simulink model "Vorlage_Anlagenteil_Pruefen_Jaehocha"  (R2021b)
settings: Solver=ode3  StartTime=0.0  StopTime=50  FixedStep=0.01  RelTol=1e-3
StopFcn:
  | clear con
model workspace (MAT data in the model file):
  A = Simulink.Signal
  A.DataType = 'auto'
  A.Dimensions = 1
  A.DimensionsMode = 'auto'
  A.Complexity = 'auto'
  A.SampleTime = -1
  A.SamplingMode = 'auto'
undefined symbols (not defined in the file): sigbuilder_block
libraries: simulink x10, simulink_extras x7, aerolibanimutils x1
(part 1 of 2)
settings Model: Creator=Jan  LastModifiedBy=mwjae
settings SolverCC: AlgebraicLoopSolver=TrustRegion
settings DataIOCC: ReturnWorkspaceOutputs=off
settings DebuggingCC: SFMachineParentedDataDiag=warning  ArithmeticOperatorsInVariantConditions=warning
settings SFSimCC: SimUseLocalCustomCode=off  CustomCodeUndefinedFunction=UseInterfaceOnly
settings RTWCC: RTWUseLocalCustomCode=off
settings CodeAppCC: StateflowObjectComments=on
settings SimscapeCC: SimscapeNormalizeSystem=off

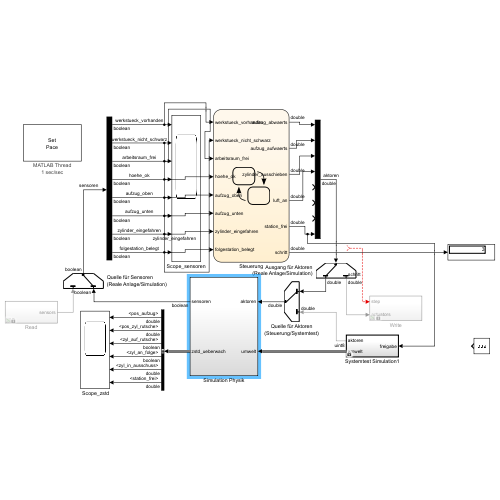
[thumbnail: Simulink's stored preview of the top-level diagram]
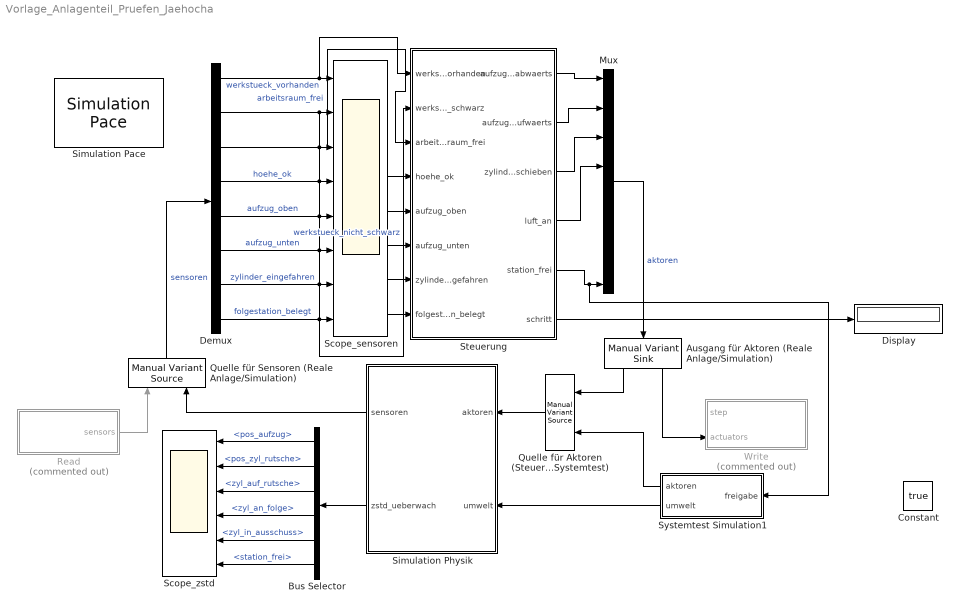
== system Vorlage_Anlagenteil_Pruefen_Jaehocha ==
  " Scope_zstd" : Scope  NumInputPorts=6
  Ausgang für Aktoren (Reale Anlage/Simulation) : simulink/Signal Routing/Manual Variant Sink  NumChoices=2  LabelModeActiveChoice=V_1
  Bus Selector : BusSelector  OutputSignals=pos_aufzug,pos_zyl_rutsche,zyl_auf_rutsche,zyl_an_folge,zyl_in_ausschuss,station_frei
  Constant : Constant  Value=true
  Demux : Demux  Outputs=8
  Display : Display
  Mux : Mux  Inputs=8
  Quelle für Aktoren (Steuerung/Systemtest) : simulink/Signal Routing/Manual Variant Source  NumChoices=2  LabelModeActiveChoice=V_1
  Quelle für Sensoren (Reale Anlage/Simulation) : simulink/Signal Routing/Manual Variant Source  NumChoices=2  LabelModeActiveChoice=V_2
  Read : Subsystem  Commented=on
  Scope_sensoren : Scope  NumInputPorts=8
  Simulation Pace : aerolibanimutils/Simulation Pace  SimulationPace=1  SleepMode=MATLAB Thread  OutputPaceError=off  SampleTime=-1
  Simulation Physik : Subsystem
  Steuerung : Stateflow chart  TreatAsAtomicUnit=on
  Systemtest Simulation1 : Subsystem  TreatAsAtomicUnit=on
  Write : Subsystem  Commented=on
  wires:
  Quelle für Sensoren (Reale Anlage/Simulation)/1 -> Demux/1  "sensoren"
  Read/1(sensors) -> Quelle für Sensoren (Reale Anlage/Simulation)/1
  Mux/1 -> Ausgang für Aktoren (Reale Anlage/Simulation)/1  "aktoren"
  Simulation Physik/1(sensoren) -> Quelle für Sensoren (Reale Anlage/Simulation)/2
  Ausgang für Aktoren (Reale Anlage/Simulation)/2 -> Write/2(actuators)
  Ausgang für Aktoren (Reale Anlage/Simulation)/1 -> Quelle für Aktoren (Steuerung/Systemtest)/1
  Quelle für Aktoren (Steuerung/Systemtest)/1 -> Simulation Physik/1(aktoren)
  Systemtest Simulation1/1(aktoren) -> Quelle für Aktoren (Steuerung/Systemtest)/2
  Systemtest Simulation1/2(umwelt) -> Simulation Physik/2(umwelt)
  Simulation Physik/2(zstd_ueberwach) -> Bus Selector/1
  Bus Selector/1 -> " Scope_zstd"/1  "<pos_aufzug>"
  Bus Selector/2 -> " Scope_zstd"/2  "<pos_zyl_rutsche>"
  Bus Selector/3 -> " Scope_zstd"/3  "<zyl_auf_rutsche>"
  Bus Selector/4 -> " Scope_zstd"/4  "<zyl_an_folge>"
  Bus Selector/5 -> " Scope_zstd"/5  "<zyl_in_ausschuss>"
  Bus Selector/6 -> " Scope_zstd"/6  "<station_frei>"
  Demux/1 -> Steuerung/1(werkstueck_vorhanden), Scope_sensoren/1  "werkstueck_vorhanden"
  Demux/2 -> Steuerung/2(werkstueck_nicht_schwarz), Scope_sensoren/2  "werkstueck_nicht_schwarz"
  Demux/3 -> Steuerung/3(arbeitsraum_frei), Scope_sensoren/3  "arbeitsraum_frei"
  Demux/4 -> Scope_sensoren/4, Steuerung/4(hoehe_ok)  "hoehe_ok"
  Demux/5 -> Steuerung/5(aufzug_oben), Scope_sensoren/5  "aufzug_oben"
  Demux/6 -> Steuerung/6(aufzug_unten), Scope_sensoren/6  "aufzug_unten"
  Demux/7 -> Steuerung/7(zylinder_eingefahren), Scope_sensoren/7  "zylinder_eingefahren"
  Demux/8 -> Steuerung/8(folgestation_belegt), Scope_sensoren/8  "folgestation_belegt"
  ? -> Write/1(step)  "schritt"
  Steuerung/5(station_frei) -> Systemtest Simulation1/1(freigabe), Mux/8
  Steuerung/1(aufzug_abwaerts) -> Mux/1
  Steuerung/2(aufzug_aufwaerts) -> Mux/2
  Steuerung/3(zylinder_ausschieben) -> Mux/3
  Steuerung/4(luft_an) -> Mux/4
  Steuerung/6(schritt) -> Display/1

== system Vorlage_Anlagenteil_Pruefen_Jaehocha/Read ==
  Read : MATLAB Function  TreatAsAtomicUnit=on
  sensors : Outport  VectorParamsAs1DForOutWhenUnconnected=off
  wires:
  Read/1(senarr) -> sensors/1

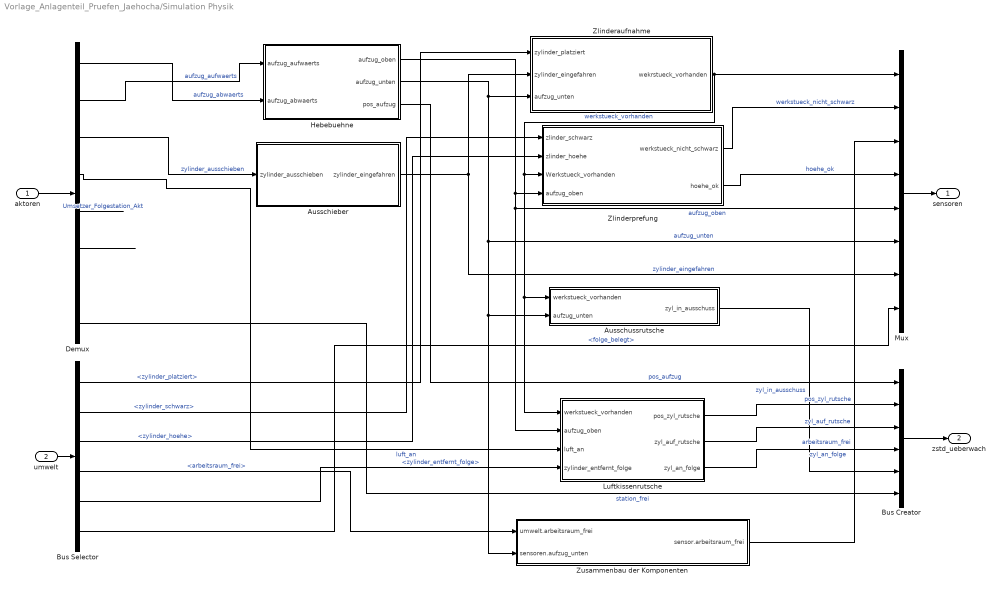
== system Vorlage_Anlagenteil_Pruefen_Jaehocha/Simulation Physik ==
  aktoren : Inport
  umwelt : Inport  Port=2
  Ausschieber : Subsystem
  Ausschussrutsche : Subsystem
  Bus Creator : BusCreator  Inputs=6
  Bus Selector : BusSelector  OutputSignals=zylinder_platziert,zylinder_schwarz,zylinder_hoehe,arbeitsraum_frei,zylinder_entfernt_folge,folge_belegt
  Demux : Demux  Outputs=8
  Hebebuehne : Subsystem
  Luftkissenrutsche : Subsystem
  Mux : Mux  Inputs=8
  Zlinderaufnahme : Subsystem
  Zlinderprefung : Subsystem
  Zusammenbau der Komponenten : Subsystem
  sensoren : Outport  VectorParamsAs1DForOutWhenUnconnected=off
  zstd_ueberwach : Outport  Port=2  VectorParamsAs1DForOutWhenUnconnected=off
  wires:
  aktoren/1 -> Demux/1
  Mux/1 -> sensoren/1
  Zusammenbau der Komponenten/1(sensor.arbeitsraum_frei) -> Mux/3  "arbeitsraum_frei"
  Demux/3 -> Ausschieber/1(zylinder_ausschieben)  "zylinder_ausschieben"
  Zlinderaufnahme/1(wekrstueck_vorhanden) -> Ausschussrutsche/1(werkstueck_vorhanden), Luftkissenrutsche/1(werkstueck_vorhanden), Zlinderprefung/3(Werkstueck_vorhanden), Mux/1  "werkstueck_vorhanden"
  Zlinderprefung/2(hoehe_ok) -> Mux/4  "hoehe_ok"
  Zlinderprefung/1(werkstueck_nicht_schwarz) -> Mux/2  "werkstueck_nicht_schwarz"
  umwelt/1 -> Bus Selector/1
  Bus Selector/2 -> Zlinderprefung/1(zlinder_schwarz)  "<zylinder_schwarz>"
  Bus Selector/4 -> Zusammenbau der Komponenten/1(umwelt.arbeitsraum_frei)  "<arbeitsraum_frei>"
  Bus Selector/5 -> Luftkissenrutsche/4(zylinder_entfernt_folge)  "<zylinder_entfernt_folge>"
  Bus Selector/6 -> Mux/8  "<folge_belegt>"
  Hebebuehne/3(pos_aufzug) -> Bus Creator/1  "pos_aufzug"
  Bus Creator/1 -> zstd_ueberwach/1
  Luftkissenrutsche/1(pos_zyl_rutsche) -> Bus Creator/2  "pos_zyl_rutsche"
  Luftkissenrutsche/2(zyl_auf_rutsche) -> Bus Creator/3  "zyl_auf_rutsche"
  Luftkissenrutsche/3(zyl_an_folge) -> Bus Creator/4  "zyl_an_folge"
  Ausschussrutsche/1(zyl_in_ausschuss) -> Bus Creator/5  "zyl_in_ausschuss"
  Hebebuehne/2(aufzug_unten) -> Mux/6, Zusammenbau der Komponenten/2(sensoren.aufzug_unten), Ausschussrutsche/2(aufzug_unten), Zlinderaufnahme/3(aufzug_unten)  "aufzug_unten"
  Ausschieber/1(zylinder_eingefahren) -> Zlinderaufnahme/2(zylinder_eingefahren), Mux/7  "zylinder_eingefahren"
  Hebebuehne/1(aufzug_oben) -> Zlinderprefung/4(aufzug_oben), Mux/5, Luftkissenrutsche/2(aufzug_oben)  "aufzug_oben"
  Bus Selector/3 -> Zlinderprefung/2(zlinder_hoehe)  "<zylinder_hoehe>"
  Demux/8 -> Bus Creator/6  "station_frei"
  Demux/1 -> Hebebuehne/2(aufzug_abwaerts)  "aufzug_abwaerts"
  Demux/2 -> Hebebuehne/1(aufzug_aufwaerts)  "aufzug_aufwaerts"
  Bus Selector/1 -> Zlinderaufnahme/1(zylinder_platziert)  "<zylinder_platziert>"
  Demux/4 -> Luftkissenrutsche/3(luft_an)  "luft_an"
  Demux/5 -> ?  "Umsetzer_Folgestation_Akt"
  Demux/6 -> ?

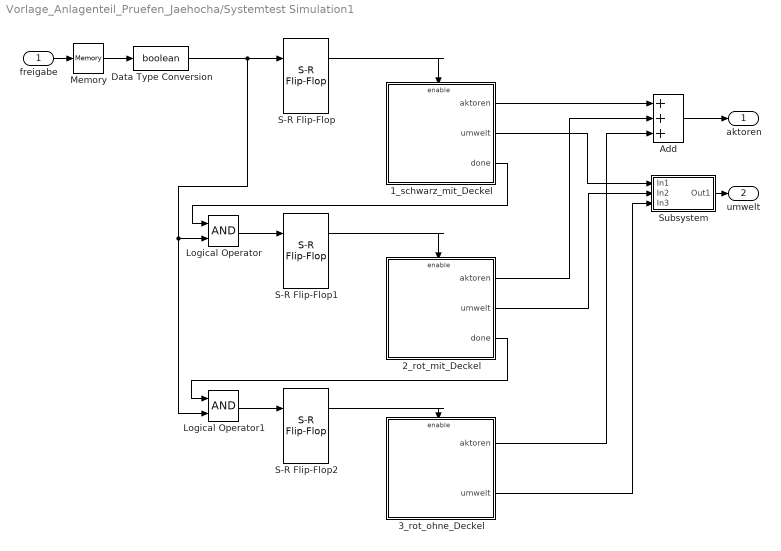
== system Vorlage_Anlagenteil_Pruefen_Jaehocha/Systemtest Simulation1 ==
  freigabe : Inport
  1_schwarz_mit_Deckel : Subsystem
  2_rot_mit_Deckel : Subsystem
  3_rot_ohne_Deckel : Subsystem
  Add : Sum  Inputs=+++
  Data Type Conversion : DataTypeConversion  OutDataTypeStr=boolean
  Logical Operator : Logic  AllPortsSameDT=off  OutDataTypeStr=boolean
  Logical Operator1 : Logic  AllPortsSameDT=off  OutDataTypeStr=boolean
  Memory : Memory
  S-R Flip-Flop : simulink_extras/Flip Flops/S-R Flip-Flop  initial_condition=0
  S-R Flip-Flop1 : simulink_extras/Flip Flops/S-R Flip-Flop  initial_condition=0
  S-R Flip-Flop2 : simulink_extras/Flip Flops/S-R Flip-Flop  initial_condition=0
  Subsystem : Subsystem
  aktoren : Outport  VectorParamsAs1DForOutWhenUnconnected=off
  umwelt : Outport  Port=2  VectorParamsAs1DForOutWhenUnconnected=off
  wires:
  freigabe/1 -> Memory/1
  S-R Flip-Flop/1 -> 1_schwarz_mit_Deckel/Enable
  Logical Operator/1 -> S-R Flip-Flop1/1
  1_schwarz_mit_Deckel/3(done) -> Logical Operator/1
  S-R Flip-Flop1/1 -> 2_rot_mit_Deckel/Enable
  Logical Operator1/1 -> S-R Flip-Flop2/1
  2_rot_mit_Deckel/3(done) -> Logical Operator1/1
  S-R Flip-Flop2/1 -> 3_rot_ohne_Deckel/Enable
  1_schwarz_mit_Deckel/1(aktoren) -> Add/1
  2_rot_mit_Deckel/1(aktoren) -> Add/2
  Add/1 -> aktoren/1
  3_rot_ohne_Deckel/1(aktoren) -> Add/3
  Subsystem/1(Out1) -> umwelt/1
  1_schwarz_mit_Deckel/2(umwelt) -> Subsystem/1(In1)
  2_rot_mit_Deckel/2(umwelt) -> Subsystem/2(In2)
  3_rot_ohne_Deckel/2(umwelt) -> Subsystem/3(In3)
  Data Type Conversion/1 -> Logical Operator1/2, Logical Operator/2, S-R Flip-Flop/1
  Memory/1 -> Data Type Conversion/1

== system Vorlage_Anlagenteil_Pruefen_Jaehocha/Write ==
  step : Inport
  actuators : Inport  Port=2
  Data Type Conversion : DataTypeConversion  OutDataTypeStr=boolean
  Write1 : MATLAB Function  TreatAsAtomicUnit=on
  wires:
  step/1 -> Write1/1(step)
  Data Type Conversion/1 -> Write1/2(actuators)
  actuators/1 -> Data Type Conversion/1

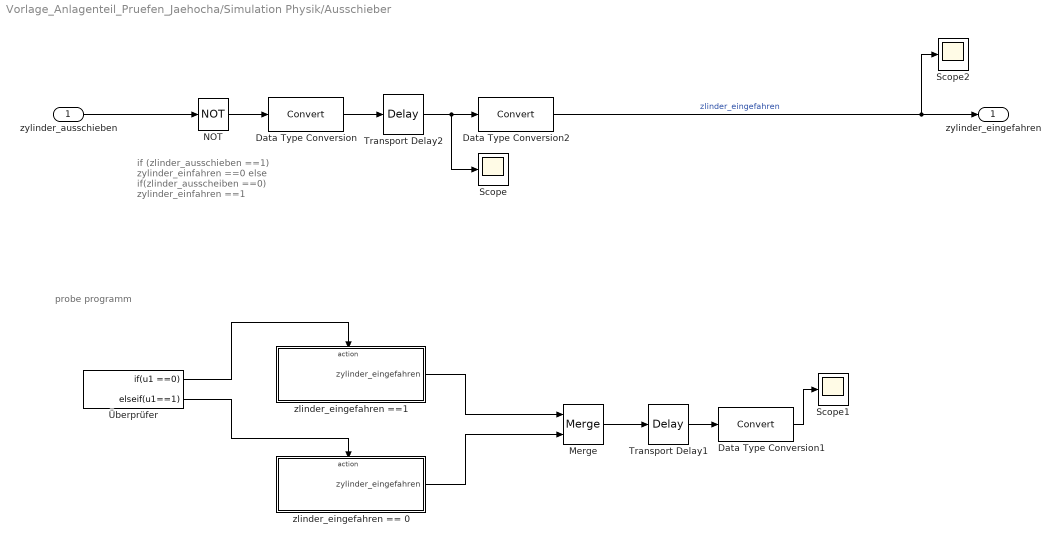
== system Vorlage_Anlagenteil_Pruefen_Jaehocha/Simulation Physik/Ausschieber ==
  note: probe programm
  note: if (zlinder_ausschieben ==1)
      |  zylinder_einfahren ==0
      | else if(zlinder_ausscheiben ==0)
      | zylinder_einfahren ==1
  zylinder_ausschieben : Inport
  Data Type Conversion : DataTypeConversion
  Data Type Conversion1 : DataTypeConversion
  Data Type Conversion2 : DataTypeConversion
  Merge : Merge
  NOT : Logic  Operator=NOT  IconShape=distinctive  AllPortsSameDT=off  OutDataTypeStr=boolean
  Scope : Scope
  Scope1 : Scope
  Scope2 : Scope
  Transport Delay1 : TransportDelay  DelayTime=0.5
  Transport Delay2 : TransportDelay  DelayTime=0.5
  zlinder_eingefahren == 0 : Subsystem  TreatAsAtomicUnit=on
  zlinder_eingefahren ==1 : Subsystem  TreatAsAtomicUnit=on
  Überprüfer : If  IfExpression=u1 ==0  ElseIfExpressions=u1==1  ShowElse=off
  zylinder_eingefahren : Outport
  wires:
  Data Type Conversion/1 -> Transport Delay2/1
  NOT/1 -> Data Type Conversion/1
  Transport Delay2/1 -> Data Type Conversion2/1, Scope/1
  zylinder_ausschieben/1 -> NOT/1
  Data Type Conversion2/1 -> zylinder_eingefahren/1, Scope2/1  "zlinder_eingefahren"
  Data Type Conversion1/1 -> Scope1/1
  zlinder_eingefahren ==1/1(zylinder_eingefahren) -> Merge/1
  Transport Delay1/1 -> Data Type Conversion1/1
  Überprüfer/2 -> zlinder_eingefahren == 0/Action
  zlinder_eingefahren == 0/1(zylinder_eingefahren) -> Merge/2
  Merge/1 -> Transport Delay1/1
  Überprüfer/1 -> zlinder_eingefahren ==1/Action

== system Vorlage_Anlagenteil_Pruefen_Jaehocha/Simulation Physik/Ausschussrutsche ==
  werkstueck_vorhanden : Inport
  aufzug_unten : Inport  Port=2
  AND : Logic  IconShape=distinctive  AllPortsSameDT=off  OutDataTypeStr=boolean
  Relational Operator : RelationalOperator  Operator=<  OutDataTypeStr=boolean  RndMeth=Simplest
  Scope : Scope  NumInputPorts=4
  Scope1 : Scope
  Triggered Subsystem for Rising edge counter : Subsystem  TreatAsAtomicUnit=on
  Unit Delay : UnitDelay  SampleTime=-1  HasFrameUpgradeWarning=on
  zyl_in_ausschuss : Outport
  wires:
  werkstueck_vorhanden/1 -> Unit Delay/1, Scope/1, Relational Operator/1  "werkstueck_vorhanden"
  aufzug_unten/1 -> Scope/3, AND/2  "aufzug_unten"
  Unit Delay/1 -> Relational Operator/2
  Relational Operator/1 -> Scope/2, AND/1  "falling Edge"
  AND/1 -> Triggered Subsystem for Rising edge counter/Trigger, Scope/4  "AND"
  Triggered Subsystem for Rising edge counter/1(zyl_in_ausschuss) -> Scope1/1, zyl_in_ausschuss/1  "zyl_in_ausschuss"

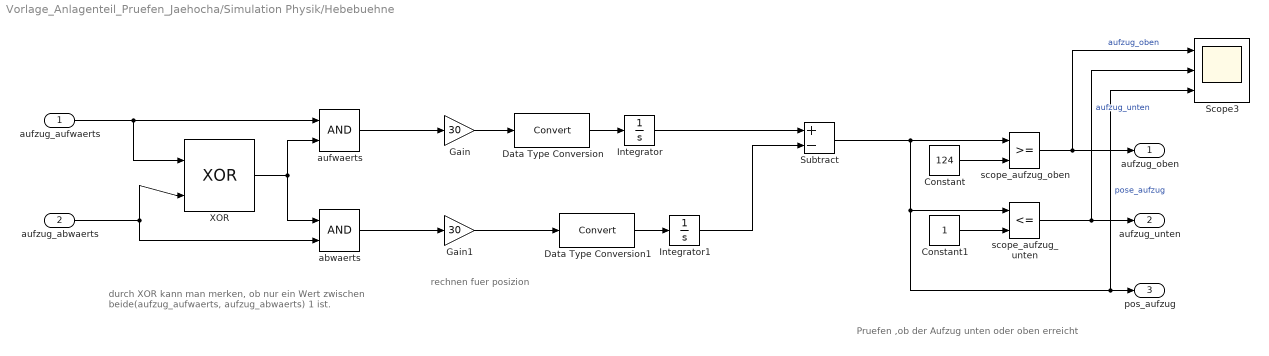
== system Vorlage_Anlagenteil_Pruefen_Jaehocha/Simulation Physik/Hebebuehne ==
  note: rechnen fuer posizion
  note: durch XOR kann man merken, ob nur ein Wert zwischen beide(aufzug_aufwaerts, aufzug_abwaerts) 1 ist.
  note: Pruefen ,ob der Aufzug unten oder oben erreicht
  aufzug_aufwaerts : Inport
  aufzug_abwaerts : Inport  Port=2
  Constant : Constant  Value=124
  Constant1 : Constant
  Data Type Conversion : DataTypeConversion
  Data Type Conversion1 : DataTypeConversion
  Gain : Gain  Gain=30
  Gain1 : Gain  Gain=30
  Integrator : Integrator  UpperSaturationLimit=125  LowerSaturationLimit=0
  Integrator1 : Integrator  UpperSaturationLimit=0  LowerSaturationLimit=-125
  Scope3 : Scope  NumInputPorts=3
  Subtract : Sum  Inputs=+-
  XOR : Logic  Operator=XOR  IconShape=distinctive  AllPortsSameDT=off  OutDataTypeStr=boolean
  abwaerts : Logic  IconShape=distinctive  AllPortsSameDT=off  OutDataTypeStr=boolean
  aufwaerts : Logic  IconShape=distinctive  AllPortsSameDT=off  OutDataTypeStr=boolean
  scope_aufzug_oben : RelationalOperator  OutDataTypeStr=boolean  RndMeth=Simplest
  scope_aufzug_unten : RelationalOperator  Operator=<=  OutDataTypeStr=boolean  RndMeth=Simplest
  aufzug_oben : Outport
  aufzug_unten : Outport  Port=2
  pos_aufzug : Outport  Port=3
  wires:
  aufzug_aufwaerts/1 -> aufwaerts/1, XOR/1
  aufzug_abwaerts/1 -> abwaerts/2, XOR/2
  XOR/1 -> abwaerts/1, aufwaerts/2
  aufwaerts/1 -> Gain/1
  abwaerts/1 -> Gain1/1
  Gain1/1 -> Data Type Conversion1/1
  Gain/1 -> Data Type Conversion/1
  Data Type Conversion/1 -> Integrator/1
  Data Type Conversion1/1 -> Integrator1/1
  Subtract/1 -> scope_aufzug_oben/1, Scope3/3, pos_aufzug/1, scope_aufzug_unten/1  "pose_aufzug"
  Integrator/1 -> Subtract/1
  scope_aufzug_oben/1 -> Scope3/1, aufzug_oben/1  "aufzug_oben"
  Constant/1 -> scope_aufzug_oben/2
  Constant1/1 -> scope_aufzug_unten/2
  scope_aufzug_unten/1 -> aufzug_unten/1, Scope3/2  "aufzug_unten"
  Integrator1/1 -> Subtract/2

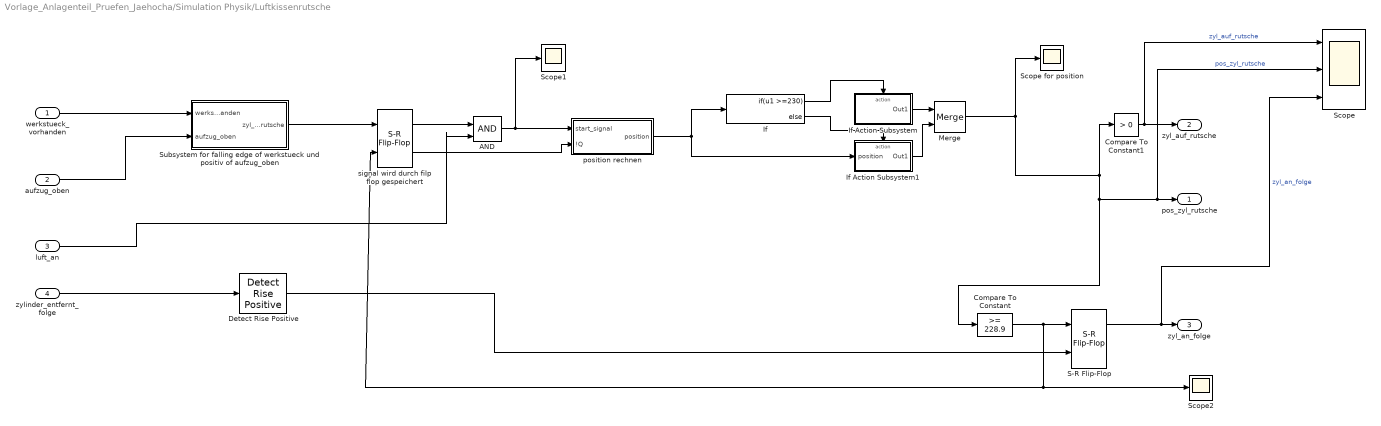
== system Vorlage_Anlagenteil_Pruefen_Jaehocha/Simulation Physik/Luftkissenrutsche ==
  werkstueck_vorhanden : Inport
  aufzug_oben : Inport  Port=2
  luft_an : Inport  Port=3
  zylinder_entfernt_folge : Inport  Port=4
  AND : Logic  IconShape=distinctive  AllPortsSameDT=off  OutDataTypeStr=boolean
  Compare To Constant : simulink/Logic and Bit Operations/Compare To Constant  relop=>=  const=228.9  OutDataTypeStr=boolean
  Compare To Constant1 : simulink/Logic and Bit Operations/Compare To Constant  relop=>  const=0  OutDataTypeStr=boolean
  Detect Rise Positive : simulink/Logic and Bit Operations/Detect Rise Positive  vinit=0  OutDataTypeStr=boolean
  If : If  IfExpression=u1 >=230
  If Action Subsystem : Subsystem  TreatAsAtomicUnit=on
  If Action Subsystem1 : Subsystem  TreatAsAtomicUnit=on
  Merge : Merge
  S-R Flip-Flop : simulink_extras/Flip Flops/S-R Flip-Flop  initial_condition=0
  Scope : Scope  NumInputPorts=3
  "Scope for position " : Scope
  Scope1 : Scope
  Scope2 : Scope
  Subsystem for falling edge of werkstueck und positiv of aufzug_oben : Subsystem
  position rechnen : Subsystem
  signal wird durch filp flop gespeichert : simulink_extras/Flip Flops/S-R Flip-Flop  initial_condition=0
  pos_zyl_rutsche : Outport
  zyl_auf_rutsche : Outport  Port=2
  zyl_an_folge : Outport  Port=3
  wires:
  werkstueck_vorhanden/1 -> Subsystem for falling edge of werkstueck und positiv of aufzug_oben/1(werkstueck_vorhanden)
  aufzug_oben/1 -> Subsystem for falling edge of werkstueck und positiv of aufzug_oben/2(aufzug_oben)
  Subsystem for falling edge of werkstueck und positiv of aufzug_oben/1(zyl_steht_auf_rutsche) -> signal wird durch filp flop gespeichert/1
  luft_an/1 -> AND/2
  zylinder_entfernt_folge/1 -> Detect Rise Positive/1
  position rechnen/1(position) -> If Action Subsystem1/1(position), If/1
  If/2 -> If Action Subsystem1/Action
  If Action Subsystem/1(Out1) -> Merge/1
  If Action Subsystem1/1(Out1) -> Merge/2
  Merge/1 -> Scope/2, pos_zyl_rutsche/1, Compare To Constant/1, Compare To Constant1/1, "Scope for position "/1  "pos_zyl_rutsche"
  Compare To Constant/1 -> Scope2/1, signal wird durch filp flop gespeichert/2, S-R Flip-Flop/1
  Detect Rise Positive/1 -> S-R Flip-Flop/2
  S-R Flip-Flop/1 -> Scope/3, zyl_an_folge/1  "zyl_an_folge"
  Compare To Constant1/1 -> Scope/1, zyl_auf_rutsche/1  "zyl_auf_rutsche"
  If/1 -> If Action Subsystem/Action
  signal wird durch filp flop gespeichert/1 -> AND/1
  AND/1 -> Scope1/1, position rechnen/1(start_signal)
  signal wird durch filp flop gespeichert/2 -> position rechnen/2(!Q)

== system Vorlage_Anlagenteil_Pruefen_Jaehocha/Simulation Physik/Zlinderaufnahme ==
  zylinder_platziert : Inport
  zylinder_eingefahren : Inport  Port=2
  aufzug_unten : Inport  Port=3
  AND : Logic  IconShape=distinctive  AllPortsSameDT=off  OutDataTypeStr=boolean
  AND1 : Logic  IconShape=distinctive  AllPortsSameDT=off  OutDataTypeStr=boolean
  Detect Fall Nonpositive : simulink/Logic and Bit Operations/Detect Fall Nonpositive  vinit=0  OutDataTypeStr=boolean
      settings: SourceProductBaseCode=SL
  Detect Rise Positive : simulink/Logic and Bit Operations/Detect Rise Positive  vinit=0  OutDataTypeStr=boolean
  S-R Flip-Flop : simulink_extras/Flip Flops/S-R Flip-Flop  initial_condition=0
  wekrstueck_vorhanden : Outport
  wires:
  zylinder_platziert/1 -> Detect Rise Positive/1
  zylinder_eingefahren/1 -> Detect Fall Nonpositive/1, AND/1
  aufzug_unten/1 -> AND/2
  Detect Rise Positive/1 -> AND1/1
  Detect Fall Nonpositive/1 -> S-R Flip-Flop/2
  S-R Flip-Flop/1 -> wekrstueck_vorhanden/1
  AND/1 -> AND1/2
  AND1/1 -> S-R Flip-Flop/1

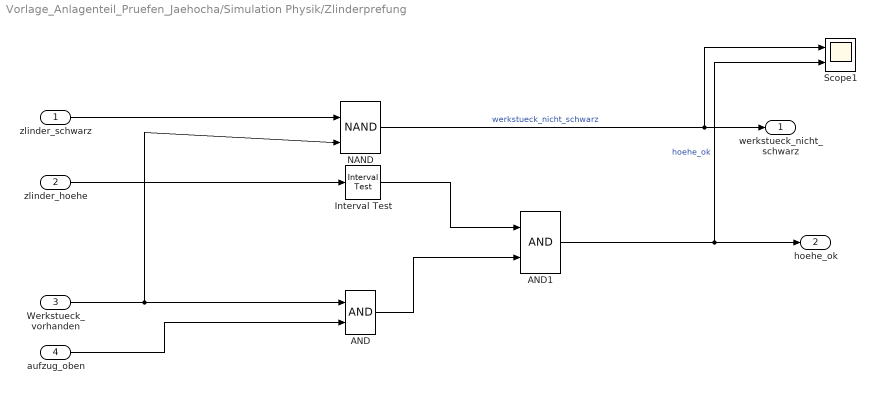
== system Vorlage_Anlagenteil_Pruefen_Jaehocha/Simulation Physik/Zlinderprefung ==
  zlinder_schwarz : Inport
  zlinder_hoehe : Inport  Port=2
  Werkstueck_vorhanden : Inport  Port=3
  aufzug_oben : Inport  Port=4
  AND : Logic  IconShape=distinctive  AllPortsSameDT=off  OutDataTypeStr=boolean
  AND1 : Logic  IconShape=distinctive  AllPortsSameDT=off  OutDataTypeStr=boolean
  Interval Test : simulink/Logic and Bit Operations/Interval Test  IntervalClosedRight=on  uplimit=26  IntervalClosedLeft=on  lowlimit=24  OutDataTypeStr=boolean
  NAND : Logic  Operator=NAND  IconShape=distinctive  AllPortsSameDT=off  OutDataTypeStr=boolean
  Scope1 : Scope  NumInputPorts=2
  werkstueck_nicht_schwarz : Outport
  hoehe_ok : Outport  Port=2
  wires:
  zlinder_schwarz/1 -> NAND/1
  Werkstueck_vorhanden/1 -> NAND/2, AND/1
  NAND/1 -> werkstueck_nicht_schwarz/1, Scope1/1  "werkstueck_nicht_schwarz"
  zlinder_hoehe/1 -> Interval Test/1
  aufzug_oben/1 -> AND/2
  Interval Test/1 -> AND1/1
  AND/1 -> AND1/2
  AND1/1 -> hoehe_ok/1, Scope1/2  "hoehe_ok"

== system Vorlage_Anlagenteil_Pruefen_Jaehocha/Simulation Physik/Zusammenbau der Komponenten ==
  umwelt.arbeitsraum_frei : Inport
  sensoren.aufzug_unten : Inport  Port=2
  AND : Logic  IconShape=distinctive  AllPortsSameDT=off  OutDataTypeStr=boolean
  sensor.arbeitsraum_frei : Outport
  wires:
  umwelt.arbeitsraum_frei/1 -> AND/1
  sensoren.aufzug_unten/1 -> AND/2
  AND/1 -> sensor.arbeitsraum_frei/1

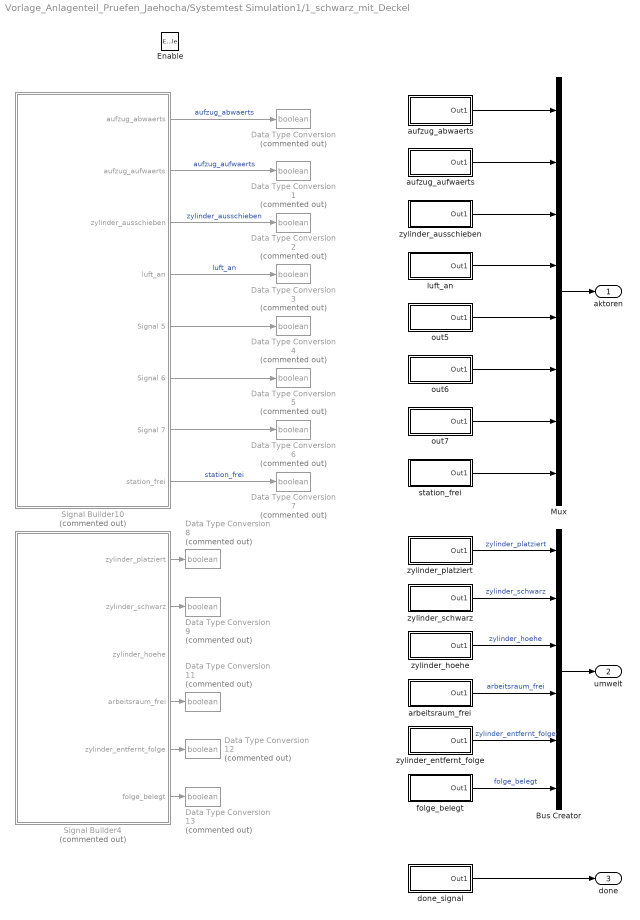
== system Vorlage_Anlagenteil_Pruefen_Jaehocha/Systemtest Simulation1/1_schwarz_mit_Deckel ==
  Enable : EnablePort
  Bus Creator : BusCreator  Inputs=6
  Data Type Conversion{,1..9,11..13} (13 alike) : DataTypeConversion  Commented=on  OutDataTypeStr=boolean
  Mux : Mux  Inputs=8
  Signal Builder10 : Subsystem  Tag=STV Subsys  Commented=on  LoadFcn=sigbuilder_block('load');  StartFcn=sigbuilder_block('start');  StopFcn=sigbuilder_block('stop');  ClipboardFcn=sigbuilder_block('clipboard');  mask(Sigbuilder block){tuvar=[0:10]}
      mask help: Simulink:masks:SigbuilderBlock_MD
      mask init:
      | if ~strcmp(get_param(bdroot(gcbh),'SimulationStatus'),'stopped') tuvar = sigbuilder_block('maskInit'); end
      settings: CopyFcn=sigbuilder_block('copy');  DeleteFcn=sigbuilder_block('delete');  ModelCloseFcn=sigbuilder_block('modelClose');  PreSaveFcn=sigbuilder_block('preSave');  PauseFcn=sigbuilder_block('pause');  ContinueFcn=sigbuilder_block('continue');  NameChangeFcn=sigbuilder_block('namechange');  OpenFcn=sigbuilder_block('open',[2160 -195 1440 817.5 ]);  CloseFcn=sigbuilder_block('close');
      mask Display: plot(0, 0, 100, 100,[2, 2, 32, 32, 2], [68, 8, 8, 68, 68],[32, 2], [38, 38], [32, 19, 2],[53, 60, 44], [32, 17, 17, 2],[16, 16, 31, 31]);txt = getActiveGroup(gcbh);text(2, 100, txt,'verticalAlignment', 'top');
  Signal Builder4 : Subsystem  Tag=STV Subsys  Commented=on  LoadFcn=sigbuilder_block('load');  StartFcn=sigbuilder_block('start');  StopFcn=sigbuilder_block('stop');  ClipboardFcn=sigbuilder_block('clipboard');  mask(Sigbuilder block){tuvar=[0:10]}
      mask help: Simulink:masks:SigbuilderBlock_MD
      mask init:
      | if ~strcmp(get_param(bdroot(gcbh),'SimulationStatus'),'stopped') tuvar = sigbuilder_block('maskInit'); end
      settings: CopyFcn=sigbuilder_block('copy');  DeleteFcn=sigbuilder_block('delete');  ModelCloseFcn=sigbuilder_block('modelClose');  PreSaveFcn=sigbuilder_block('preSave');  PauseFcn=sigbuilder_block('pause');  ContinueFcn=sigbuilder_block('continue');  NameChangeFcn=sigbuilder_block('namechange');  OpenFcn=sigbuilder_block('open',[4.875 4.875 1070.25 612.75 ]);  CloseFcn=sigbuilder_block('close');
      mask Display: plot(0, 0, 100, 100,[2, 2, 32, 32, 2], [68, 8, 8, 68, 68],[32, 2], [38, 38], [32, 19, 2],[53, 60, 44], [32, 17, 17, 2],[16, 16, 31, 31]);txt = getActiveGroup(gcbh);text(2, 100, txt,'verticalAlignment', 'top');
  arbeitsraum_frei : Subsystem
  aufzug_abwaerts : Subsystem
  aufzug_aufwaerts : Subsystem
  done_signal : Subsystem
  folge_belegt : Subsystem
  luft_an : Subsystem
  out5 : Subsystem
  out6 : Subsystem
  out7 : Subsystem
  station_frei : Subsystem
  zylinder_ausschieben : Subsystem
  zylinder_entfernt_folge : Subsystem
  zylinder_hoehe : Subsystem
  zylinder_platziert : Subsystem
  zylinder_schwarz : Subsystem
  aktoren : Outport  VectorParamsAs1DForOutWhenUnconnected=off
  umwelt : Outport  Port=2  VectorParamsAs1DForOutWhenUnconnected=off
  done : Outport  Port=3  VectorParamsAs1DForOutWhenUnconnected=off
  wires:
  Bus Creator/1 -> umwelt/1
  Signal Builder4/1(zylinder_platziert) -> Data Type Conversion8/1
  Signal Builder4/2(zylinder_schwarz) -> Data Type Conversion9/1
  zylinder_hoehe/1(Out1) -> Bus Creator/3  "zylinder_hoehe"
  Signal Builder4/4(arbeitsraum_frei) -> Data Type Conversion11/1
  Signal Builder4/5(zylinder_entfernt_folge) -> Data Type Conversion12/1
  Signal Builder4/6(folge_belegt) -> Data Type Conversion13/1
  zylinder_platziert/1(Out1) -> Bus Creator/1  "zylinder_platziert"
  zylinder_schwarz/1(Out1) -> Bus Creator/2  "zylinder_schwarz"
  arbeitsraum_frei/1(Out1) -> Bus Creator/4  "arbeitsraum_frei"
  zylinder_entfernt_folge/1(Out1) -> Bus Creator/5  "zylinder_entfernt_folge"
  folge_belegt/1(Out1) -> Bus Creator/6  "folge_belegt"
  Mux/1 -> aktoren/1
  Signal Builder10/1(aufzug_abwaerts) -> Data Type Conversion/1  "aufzug_abwaerts"
  Signal Builder10/2(aufzug_aufwaerts) -> Data Type Conversion1/1  "aufzug_aufwaerts"
  Signal Builder10/3(zylinder_ausschieben) -> Data Type Conversion2/1  "zylinder_ausschieben"
  Signal Builder10/4(luft_an) -> Data Type Conversion3/1  "luft_an"
  Signal Builder10/8(station_frei) -> Data Type Conversion7/1  "station_frei"
  Signal Builder10/5(Signal 5) -> Data Type Conversion4/1
  Signal Builder10/6(Signal 6) -> Data Type Conversion5/1
  Signal Builder10/7(Signal 7) -> Data Type Conversion6/1
  aufzug_abwaerts/1(Out1) -> Mux/1
  aufzug_aufwaerts/1(Out1) -> Mux/2
  zylinder_ausschieben/1(Out1) -> Mux/3
  luft_an/1(Out1) -> Mux/4
  out5/1(Out1) -> Mux/5
  out6/1(Out1) -> Mux/6
  out7/1(Out1) -> Mux/7
  station_frei/1(Out1) -> Mux/8
  done_signal/1(Out1) -> done/1

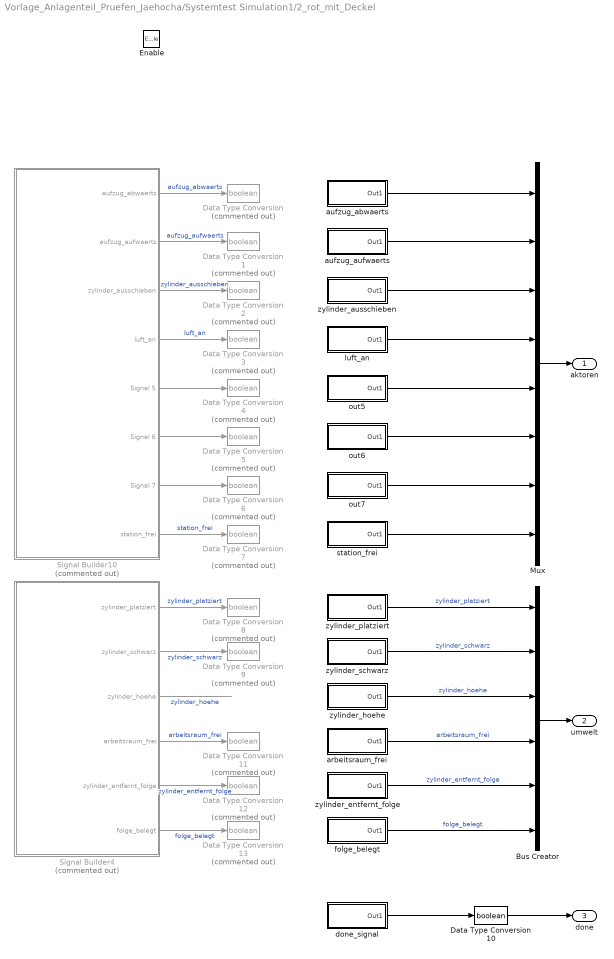
== system Vorlage_Anlagenteil_Pruefen_Jaehocha/Systemtest Simulation1/2_rot_mit_Deckel ==
  Enable : EnablePort
  Bus Creator : BusCreator  Inputs=6
  Data Type Conversion{,1..9,11..13} (13 alike) : DataTypeConversion  Commented=on  OutDataTypeStr=boolean
  Data Type Conversion10 : DataTypeConversion  OutDataTypeStr=boolean
  Mux : Mux  Inputs=8
  Signal Builder10 : Subsystem  Tag=STV Subsys  Commented=on  LoadFcn=sigbuilder_block('load');  StartFcn=sigbuilder_block('start');  StopFcn=sigbuilder_block('stop');  ClipboardFcn=sigbuilder_block('clipboard');  mask(Sigbuilder block){tuvar=[0:10]}
      mask help: Simulink:masks:SigbuilderBlock_MD
      mask init:
      | if ~strcmp(get_param(bdroot(gcbh),'SimulationStatus'),'stopped') tuvar = sigbuilder_block('maskInit'); end
      settings: CopyFcn=sigbuilder_block('copy');  DeleteFcn=sigbuilder_block('delete');  ModelCloseFcn=sigbuilder_block('modelClose');  PreSaveFcn=sigbuilder_block('preSave');  PauseFcn=sigbuilder_block('pause');  ContinueFcn=sigbuilder_block('continue');  NameChangeFcn=sigbuilder_block('namechange');  OpenFcn=sigbuilder_block('open',[4.875 4.875 1070.25 612.75 ]);  CloseFcn=sigbuilder_block('close');
      mask Display: plot(0, 0, 100, 100,[2, 2, 32, 32, 2], [68, 8, 8, 68, 68],[32, 2], [38, 38], [32, 19, 2],[53, 60, 44], [32, 17, 17, 2],[16, 16, 31, 31]);txt = getActiveGroup(gcbh);text(2, 100, txt,'verticalAlignment', 'top');
  Signal Builder4 : Subsystem  Tag=STV Subsys  Commented=on  LoadFcn=sigbuilder_block('load');  StartFcn=sigbuilder_block('start');  StopFcn=sigbuilder_block('stop');  ClipboardFcn=sigbuilder_block('clipboard');  mask(Sigbuilder block){tuvar=[0:10]}
      mask help: Simulink:masks:SigbuilderBlock_MD
      mask init:
      | if ~strcmp(get_param(bdroot(gcbh),'SimulationStatus'),'stopped') tuvar = sigbuilder_block('maskInit'); end
      settings: CopyFcn=sigbuilder_block('copy');  DeleteFcn=sigbuilder_block('delete');  ModelCloseFcn=sigbuilder_block('modelClose');  PreSaveFcn=sigbuilder_block('preSave');  PauseFcn=sigbuilder_block('pause');  ContinueFcn=sigbuilder_block('continue');  NameChangeFcn=sigbuilder_block('namechange');  OpenFcn=sigbuilder_block('open',[2160 -195 1440 817.5 ]);  CloseFcn=sigbuilder_block('close');
      mask Display: plot(0, 0, 100, 100,[2, 2, 32, 32, 2], [68, 8, 8, 68, 68],[32, 2], [38, 38], [32, 19, 2],[53, 60, 44], [32, 17, 17, 2],[16, 16, 31, 31]);txt = getActiveGroup(gcbh);text(2, 100, txt,'verticalAlignment', 'top');
  arbeitsraum_frei : Subsystem
  aufzug_abwaerts : Subsystem
  aufzug_aufwaerts : Subsystem
  done_signal : Subsystem
  folge_belegt : Subsystem
  luft_an : Subsystem
  out5 : Subsystem
  out6 : Subsystem
  out7 : Subsystem
  station_frei : Subsystem
  zylinder_ausschieben : Subsystem
  zylinder_entfernt_folge : Subsystem
  zylinder_hoehe : Subsystem
  zylinder_platziert : Subsystem
  zylinder_schwarz : Subsystem
  aktoren : Outport  VectorParamsAs1DForOutWhenUnconnected=off
  umwelt : Outport  Port=2  VectorParamsAs1DForOutWhenUnconnected=off
  done : Outport  Port=3  VectorParamsAs1DForOutWhenUnconnected=off
  wires:
  Bus Creator/1 -> umwelt/1
  Signal Builder4/1(zylinder_platziert) -> Data Type Conversion8/1  "zylinder_platziert"
  Signal Builder4/2(zylinder_schwarz) -> Data Type Conversion9/1  "zylinder_schwarz"
  Signal Builder4/3(zylinder_hoehe) -> ?  "zylinder_hoehe"
  Signal Builder4/4(arbeitsraum_frei) -> Data Type Conversion11/1  "arbeitsraum_frei"
  Signal Builder4/5(zylinder_entfernt_folge) -> Data Type Conversion12/1  "zylinder_entfernt_folge"
  Signal Builder4/6(folge_belegt) -> Data Type Conversion13/1  "folge_belegt"
  zylinder_platziert/1(Out1) -> Bus Creator/1  "zylinder_platziert"
  zylinder_schwarz/1(Out1) -> Bus Creator/2  "zylinder_schwarz"
  arbeitsraum_frei/1(Out1) -> Bus Creator/4  "arbeitsraum_frei"
  zylinder_entfernt_folge/1(Out1) -> Bus Creator/5  "zylinder_entfernt_folge"
  folge_belegt/1(Out1) -> Bus Creator/6  "folge_belegt"
  Mux/1 -> aktoren/1
  Signal Builder10/1(aufzug_abwaerts) -> Data Type Conversion/1  "aufzug_abwaerts"
  Signal Builder10/2(aufzug_aufwaerts) -> Data Type Conversion1/1  "aufzug_aufwaerts"
  Signal Builder10/3(zylinder_ausschieben) -> Data Type Conversion2/1  "zylinder_ausschieben"
  Signal Builder10/4(luft_an) -> Data Type Conversion3/1  "luft_an"
  Signal Builder10/8(station_frei) -> Data Type Conversion7/1  "station_frei"
  Signal Builder10/5(Signal 5) -> Data Type Conversion4/1
  Signal Builder10/6(Signal 6) -> Data Type Conversion5/1
  Signal Builder10/7(Signal 7) -> Data Type Conversion6/1
  aufzug_abwaerts/1(Out1) -> Mux/1
  aufzug_aufwaerts/1(Out1) -> Mux/2
  zylinder_ausschieben/1(Out1) -> Mux/3
  luft_an/1(Out1) -> Mux/4
  out5/1(Out1) -> Mux/5
  out6/1(Out1) -> Mux/6
  out7/1(Out1) -> Mux/7
  station_frei/1(Out1) -> Mux/8
  Data Type Conversion10/1 -> done/1
  done_signal/1(Out1) -> Data Type Conversion10/1
  zylinder_hoehe/1(Out1) -> Bus Creator/3  "zylinder_hoehe"

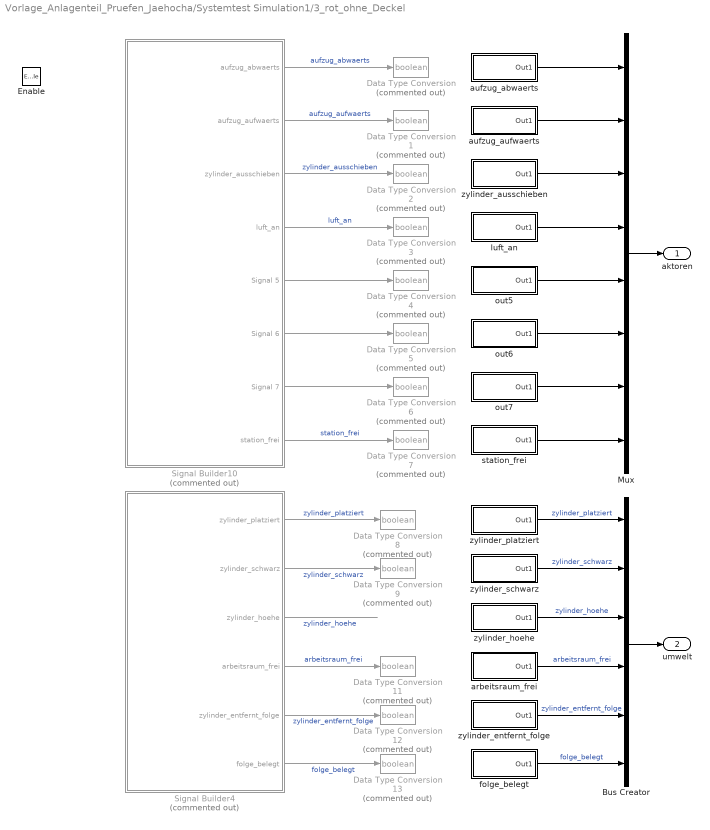
== system Vorlage_Anlagenteil_Pruefen_Jaehocha/Systemtest Simulation1/3_rot_ohne_Deckel ==
  Enable : EnablePort
  Bus Creator : BusCreator  Inputs=6
  Data Type Conversion{,1..9,11..13} (13 alike) : DataTypeConversion  Commented=on  OutDataTypeStr=boolean
  Mux : Mux  Inputs=8
  Signal Builder10 : Subsystem  Tag=STV Subsys  Commented=on  LoadFcn=sigbuilder_block('load');  StartFcn=sigbuilder_block('start');  StopFcn=sigbuilder_block('stop');  ClipboardFcn=sigbuilder_block('clipboard');  mask(Sigbuilder block){tuvar=[0:10]}
      mask help: Simulink:masks:SigbuilderBlock_MD
      mask init:
      | if ~strcmp(get_param(bdroot(gcbh),'SimulationStatus'),'stopped') tuvar = sigbuilder_block('maskInit'); end
      settings: CopyFcn=sigbuilder_block('copy');  DeleteFcn=sigbuilder_block('delete');  ModelCloseFcn=sigbuilder_block('modelClose');  PreSaveFcn=sigbuilder_block('preSave');  PauseFcn=sigbuilder_block('pause');  ContinueFcn=sigbuilder_block('continue');  NameChangeFcn=sigbuilder_block('namechange');  OpenFcn=sigbuilder_block('open',[2160 -195 1440 817.5 ]);  CloseFcn=sigbuilder_block('close');
      mask Display: plot(0, 0, 100, 100,[2, 2, 32, 32, 2], [68, 8, 8, 68, 68],[32, 2], [38, 38], [32, 19, 2],[53, 60, 44], [32, 17, 17, 2],[16, 16, 31, 31]);txt = getActiveGroup(gcbh);text(2, 100, txt,'verticalAlignment', 'top');
  Signal Builder4 : Subsystem  Tag=STV Subsys  Commented=on  LoadFcn=sigbuilder_block('load');  StartFcn=sigbuilder_block('start');  StopFcn=sigbuilder_block('stop');  ClipboardFcn=sigbuilder_block('clipboard');  mask(Sigbuilder block){tuvar=[0:10]}
      mask help: Simulink:masks:SigbuilderBlock_MD
      mask init:
      | if ~strcmp(get_param(bdroot(gcbh),'SimulationStatus'),'stopped') tuvar = sigbuilder_block('maskInit'); end
      settings: CopyFcn=sigbuilder_block('copy');  DeleteFcn=sigbuilder_block('delete');  ModelCloseFcn=sigbuilder_block('modelClose');  PreSaveFcn=sigbuilder_block('preSave');  PauseFcn=sigbuilder_block('pause');  ContinueFcn=sigbuilder_block('continue');  NameChangeFcn=sigbuilder_block('namechange');  OpenFcn=sigbuilder_block('open',[2160 -195 1440 817.5 ]);  CloseFcn=sigbuilder_block('close');
      mask Display: plot(0, 0, 100, 100,[2, 2, 32, 32, 2], [68, 8, 8, 68, 68],[32, 2], [38, 38], [32, 19, 2],[53, 60, 44], [32, 17, 17, 2],[16, 16, 31, 31]);txt = getActiveGroup(gcbh);text(2, 100, txt,'verticalAlignment', 'top');
  arbeitsraum_frei : Subsystem
  aufzug_abwaerts : Subsystem
  aufzug_aufwaerts : Subsystem
  folge_belegt : Subsystem
  luft_an : Subsystem
  out5 : Subsystem
  out6 : Subsystem
  out7 : Subsystem
  station_frei : Subsystem
  zylinder_ausschieben : Subsystem
  zylinder_entfernt_folge : Subsystem
  zylinder_hoehe : Subsystem
  zylinder_platziert : Subsystem
  zylinder_schwarz : Subsystem
  aktoren : Outport  VectorParamsAs1DForOutWhenUnconnected=off
  umwelt : Outport  Port=2  VectorParamsAs1DForOutWhenUnconnected=off
  wires:
  Bus Creator/1 -> umwelt/1
  Signal Builder4/1(zylinder_platziert) -> Data Type Conversion8/1  "zylinder_platziert"
  Signal Builder4/2(zylinder_schwarz) -> Data Type Conversion9/1  "zylinder_schwarz"
  Signal Builder4/3(zylinder_hoehe) -> ?  "zylinder_hoehe"
  Signal Builder4/4(arbeitsraum_frei) -> Data Type Conversion11/1  "arbeitsraum_frei"
  Signal Builder4/5(zylinder_entfernt_folge) -> Data Type Conversion12/1  "zylinder_entfernt_folge"
  Signal Builder4/6(folge_belegt) -> Data Type Conversion13/1  "folge_belegt"
  zylinder_platziert/1(Out1) -> Bus Creator/1  "zylinder_platziert"
  zylinder_schwarz/1(Out1) -> Bus Creator/2  "zylinder_schwarz"
  arbeitsraum_frei/1(Out1) -> Bus Creator/4  "arbeitsraum_frei"
  zylinder_entfernt_folge/1(Out1) -> Bus Creator/5  "zylinder_entfernt_folge"
  folge_belegt/1(Out1) -> Bus Creator/6  "folge_belegt"
  Mux/1 -> aktoren/1
  Signal Builder10/1(aufzug_abwaerts) -> Data Type Conversion/1  "aufzug_abwaerts"
  Signal Builder10/2(aufzug_aufwaerts) -> Data Type Conversion1/1  "aufzug_aufwaerts"
  Signal Builder10/3(zylinder_ausschieben) -> Data Type Conversion2/1  "zylinder_ausschieben"
  Signal Builder10/4(luft_an) -> Data Type Conversion3/1  "luft_an"
  Signal Builder10/8(station_frei) -> Data Type Conversion7/1  "station_frei"
  Signal Builder10/5(Signal 5) -> Data Type Conversion4/1
  Signal Builder10/6(Signal 6) -> Data Type Conversion5/1
  Signal Builder10/7(Signal 7) -> Data Type Conversion6/1
  aufzug_abwaerts/1(Out1) -> Mux/1
  aufzug_aufwaerts/1(Out1) -> Mux/2
  zylinder_ausschieben/1(Out1) -> Mux/3
  luft_an/1(Out1) -> Mux/4
  out5/1(Out1) -> Mux/5
  out6/1(Out1) -> Mux/6
  out7/1(Out1) -> Mux/7
  station_frei/1(Out1) -> Mux/8
  zylinder_hoehe/1(Out1) -> Bus Creator/3  "zylinder_hoehe"

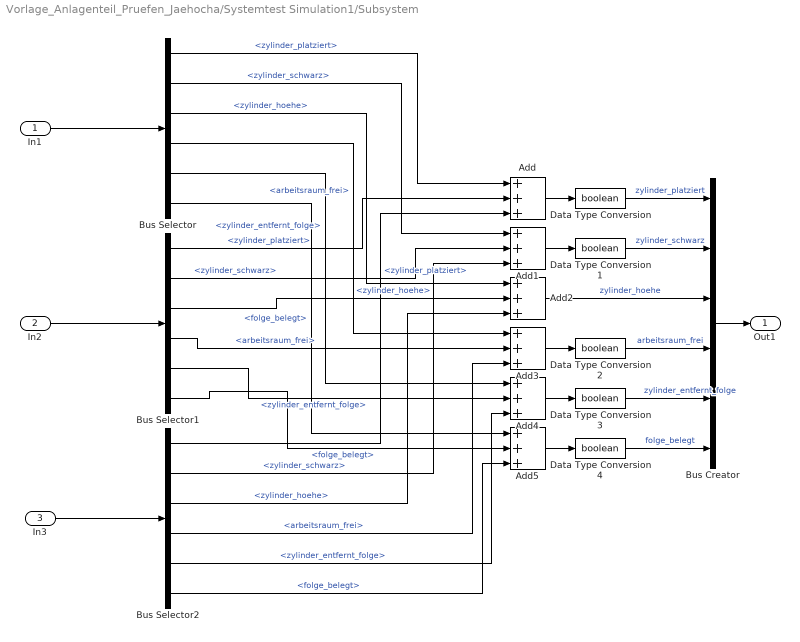
== system Vorlage_Anlagenteil_Pruefen_Jaehocha/Systemtest Simulation1/Subsystem ==
  In1 : Inport
  In2 : Inport  Port=2
  In3 : Inport  Port=3
  Add{,1..5} (6 alike) : Sum  Inputs=+++
  Bus Creator : BusCreator  Inputs=6
  Bus Selector : BusSelector  OutputSignals=zylinder_platziert,zylinder_schwarz,zylinder_hoehe,arbeitsraum_frei,zylinder_entfernt_folge,folge_belegt
  Bus Selector1 : BusSelector  OutputSignals=zylinder_platziert,zylinder_schwarz,zylinder_hoehe,arbeitsraum_frei,zylinder_entfernt_folge,folge_belegt
  Bus Selector2 : BusSelector  OutputSignals=zylinder_platziert,zylinder_schwarz,zylinder_hoehe,arbeitsraum_frei,zylinder_entfernt_folge,folge_belegt
  Data Type Conversion{,1..4} (5 alike) : DataTypeConversion  OutDataTypeStr=boolean
  Out1 : Outport  VectorParamsAs1DForOutWhenUnconnected=off
  wires:
  In1/1 -> Bus Selector/1
  In2/1 -> Bus Selector1/1
  In3/1 -> Bus Selector2/1
  Bus Creator/1 -> Out1/1
  Bus Selector/1 -> Add/1  "<zylinder_platziert>"
  Data Type Conversion/1 -> Bus Creator/1  "zylinder_platziert"
  Bus Selector1/1 -> Add/2  "<zylinder_platziert>"
  Bus Selector2/1 -> Add/3  "<zylinder_platziert>"
  Data Type Conversion1/1 -> Bus Creator/2  "zylinder_schwarz"
  Bus Selector/2 -> Add1/1  "<zylinder_schwarz>"
  Bus Selector1/2 -> Add1/2  "<zylinder_schwarz>"
  Bus Selector2/2 -> Add1/3  "<zylinder_schwarz>"
  Add2/1 -> Bus Creator/3  "zylinder_hoehe"
  Bus Selector/3 -> Add2/1  "<zylinder_hoehe>"
  Bus Selector1/3 -> Add2/2  "<zylinder_hoehe>"
  Bus Selector2/3 -> Add2/3  "<zylinder_hoehe>"
  Add3/1 -> Data Type Conversion2/1
  Bus Selector/4 -> Add3/1  "<arbeitsraum_frei>"
  Bus Selector1/4 -> Add3/2  "<arbeitsraum_frei>"
  Bus Selector2/4 -> Add3/3  "<arbeitsraum_frei>"
  Data Type Conversion3/1 -> Bus Creator/5  "zylinder_entfernt_folge"
  Bus Selector/5 -> Add4/1  "<zylinder_entfernt_folge>"
  Bus Selector1/5 -> Add4/2  "<zylinder_entfernt_folge>"
  Bus Selector2/5 -> Add4/3  "<zylinder_entfernt_folge>"
  Add5/1 -> Data Type Conversion4/1
  Bus Selector/6 -> Add5/1  "<folge_belegt>"
  Bus Selector1/6 -> Add5/2  "<folge_belegt>"
  Bus Selector2/6 -> Add5/3  "<folge_belegt>"
  Add/1 -> Data Type Conversion/1
  Add1/1 -> Data Type Conversion1/1
  Data Type Conversion2/1 -> Bus Creator/4  "arbeitsraum_frei"
  Add4/1 -> Data Type Conversion3/1
  Data Type Conversion4/1 -> Bus Creator/6  "folge_belegt"

== system Vorlage_Anlagenteil_Pruefen_Jaehocha/Simulation Physik/Ausschieber/zlinder_eingefahren == 0 ==
  Action Port : ActionPort  ActionPortLabel=elseif(u1==1)
  Constant : Constant  Value=0
  zylinder_eingefahren : Outport
  wires:
  Constant/1 -> zylinder_eingefahren/1

== system Vorlage_Anlagenteil_Pruefen_Jaehocha/Simulation Physik/Ausschieber/zlinder_eingefahren ==1 ==
  Action Port : ActionPort  ActionPortLabel=if(u1 ==0)
  Constant : Constant
  zylinder_eingefahren : Outport
  wires:
  Constant/1 -> zylinder_eingefahren/1

== system Vorlage_Anlagenteil_Pruefen_Jaehocha/Simulation Physik/Ausschussrutsche/Triggered Subsystem for Rising edge counter ==
  Trigger : TriggerPort  VariantControl=(inherit)
  Add : Sum
  Constant : Constant
  Memory : Memory  InheritSampleTime=on
  zyl_in_ausschuss : Outport
  wires:
  Add/1 -> zyl_in_ausschuss/1, Memory/1
  Constant/1 -> Add/1
  Memory/1 -> Add/2

== system Vorlage_Anlagenteil_Pruefen_Jaehocha/Simulation Physik/Luftkissenrutsche/If Action Subsystem ==
  Action Port : ActionPort  ActionPortLabel=if(u1 >=230)
  Constant : Constant  Value=0
  Out1 : Outport
  wires:
  Constant/1 -> Out1/1

== system Vorlage_Anlagenteil_Pruefen_Jaehocha/Simulation Physik/Luftkissenrutsche/If Action Subsystem1 ==
  position : Inport
  Action Port : ActionPort  ActionPortLabel=else
  Out1 : Outport
  wires:
  position/1 -> Out1/1

== system Vorlage_Anlagenteil_Pruefen_Jaehocha/Simulation Physik/Luftkissenrutsche/Subsystem for falling edge of werkstueck und positiv of aufzug_oben ==
  werkstueck_vorhanden : Inport
  aufzug_oben : Inport  Port=2
  AND : Logic  IconShape=distinctive  AllPortsSameDT=off  OutDataTypeStr=boolean
  Detect Fall Nonpositive : simulink/Logic and Bit Operations/Detect Fall Nonpositive  vinit=0  OutDataTypeStr=boolean
      settings: SourceProductBaseCode=SL
  Scope1 : Scope  NumInputPorts=3
  zyl_steht_auf_rutsche : Outport
  wires:
  werkstueck_vorhanden/1 -> Detect Fall Nonpositive/1
  Detect Fall Nonpositive/1 -> Scope1/1, AND/1
  aufzug_oben/1 -> Scope1/2, AND/2
  AND/1 -> zyl_steht_auf_rutsche/1, Scope1/3

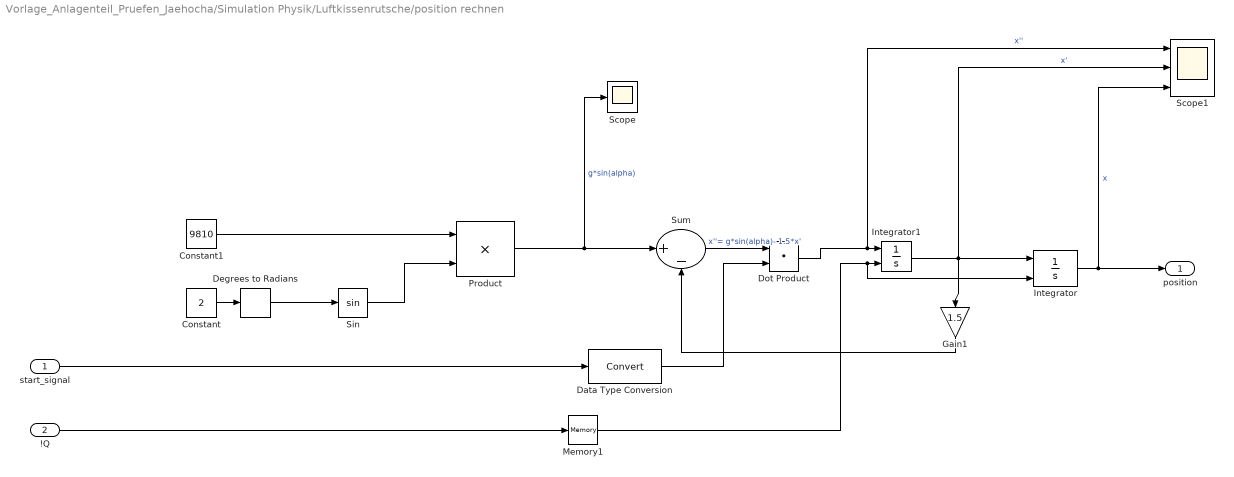
== system Vorlage_Anlagenteil_Pruefen_Jaehocha/Simulation Physik/Luftkissenrutsche/position rechnen ==
  start_signal : Inport
  !Q : Inport  Port=2
  Constant : Constant  Value=2
  Constant1 : Constant  Value=9810
  Data Type Conversion : DataTypeConversion
  Degrees to Radians : simulink_extras/Transformations/Degrees to Radians
  Dot Product : DotProduct  InputSameDT=on  OutDataTypeStr=Inherit: Inherit via internal rule
  Gain1 : Gain  Gain=1.5
  Integrator : Integrator  ExternalReset=rising  LimitOutput=on  UpperSaturationLimit=230  LowerSaturationLimit=0
  Integrator1 : Integrator  ExternalReset=rising
  Memory1 : Memory
  Product : Product
  Scope : Scope
  Scope1 : Scope  NumInputPorts=3
  Sin : Trigonometry
  Sum : Sum  Inputs=|+-
  position : Outport
  wires:
  Integrator/1 -> Scope1/3, position/1  "x"
  Integrator1/1 -> Gain1/1, Integrator/1, Scope1/2  "x'"
  Constant1/1 -> Product/1
  Degrees to Radians/1 -> Sin/1
  Constant/1 -> Degrees to Radians/1
  Product/1 -> Sum/1, Scope/1  "g*sin(alpha)"
  Sin/1 -> Product/2
  Gain1/1 -> Sum/2
  Sum/1 -> Dot Product/1  "x''= g*sin(alpha)- 1.5*x'"
  Dot Product/1 -> Scope1/1, Integrator1/1  "x''"
  Data Type Conversion/1 -> Dot Product/2
  start_signal/1 -> Data Type Conversion/1
  !Q/1 -> Memory1/1
  Memory1/1 -> Integrator/2, Integrator1/2

== system Vorlage_Anlagenteil_Pruefen_Jaehocha/Systemtest Simulation1/1_schwarz_mit_Deckel/Signal Builder10 ==
  Demux : Demux  Tag=STV Demux  Outputs=8
      settings: DisplayOption=none
  FromWs : FromWorkspace  Tag=STV FromWs  VariableName=tuvar
      SigBuilderData=|
      | common.afterFinalStr = 'Extrapolate'
      | common.sampleTime = 0
      | dataSet.timeRange = [0 11]
      | dataSet.name = 'Group 1'
      | sbobj.Groups.Name = 'Group 1'
      | sbobj.Groups.Signals(1).Name = 'aufzug_abwaerts'
      | sbobj.Groups.Signals(1).XData = [0 6 6 10.5 10.5 11]
      | sbobj.Groups.Signals(1).YData = [0 0 1 1 0 0]
      | sbobj.Groups.Signals(2).Name = 'aufzug_aufwaerts'
      | sbobj.Groups.Signals(2).XData = [0 0.5 0.5 5 5 11]
      | sbobj.Groups.Signals(2).YData = [0 0 1 1 0 0]
      | sbobj.Groups.Signals(3).Name = 'zylinder_ausschieben'
      | sbobj.Groups.Signals(3).XData = [0 5.5 5.5 6.2 6.2 11]
      | sbobj.Groups.Signals(3).YData = [0 0 1 1 0 0]
      | sbobj.Groups.Signals(4).Name = 'luft_an'
      | sbobj.Groups.Signals(4).XData = [0 5.5 5.5 7.5 7.5 11]
      | sbobj.Groups.Signals(4).YData = [0 0 1 1 0 0]
      | sbobj.Groups.Signals(5).Name = 'Signal 5'
      | sbobj.Groups.Signals(5).XData = [0 11]
      | sbobj.Groups.Signals(5).YData = [0 0]
      | sbobj.Groups.Signals(6).Name = 'Signal 6'
      | sbobj.Groups.Signals(6).XData = [0 11]
      | sbobj.Groups.Signals(6).YData = [0 0]
      | sbobj.Groups.Signals(7).Name = 'Signal 7'
      | sbobj.Groups.Signals(7).XData = [0 11]
      | sbobj.Groups.Signals(7).YData = [0 0]
      | sbobj.Groups.Signals(8).Name = 'station_frei'
      | sbobj.Groups.Signals(8).XData = [0 0.1 0.1 11]
      | sbobj.Groups.Signals(8).YData = [1 1 0 0]
      | sbobj.Groups.TimeRange = [0 11]
  aufzug_abwaerts : Outport  Tag=STV Outport  VectorParamsAs1DForOutWhenUnconnected=off
  aufzug_aufwaerts : Outport  Tag=STV Outport  Port=2  VectorParamsAs1DForOutWhenUnconnected=off
  zylinder_ausschieben : Outport  Tag=STV Outport  Port=3  VectorParamsAs1DForOutWhenUnconnected=off
  luft_an : Outport  Tag=STV Outport  Port=4  VectorParamsAs1DForOutWhenUnconnected=off
  Signal 5 : Outport  Tag=STV Outport  Port=5  VectorParamsAs1DForOutWhenUnconnected=off
  Signal 6 : Outport  Tag=STV Outport  Port=6  VectorParamsAs1DForOutWhenUnconnected=off
  Signal 7 : Outport  Tag=STV Outport  Port=7  VectorParamsAs1DForOutWhenUnconnected=off
  station_frei : Outport  Tag=STV Outport  Port=8  VectorParamsAs1DForOutWhenUnconnected=off
  wires:
  Demux/1 -> aufzug_abwaerts/1
  FromWs/1 -> Demux/1
  Demux/2 -> aufzug_aufwaerts/1
  Demux/3 -> zylinder_ausschieben/1
  Demux/4 -> luft_an/1
  Demux/5 -> Signal 5/1
  Demux/6 -> Signal 6/1
  Demux/7 -> Signal 7/1
  Demux/8 -> station_frei/1

== system Vorlage_Anlagenteil_Pruefen_Jaehocha/Systemtest Simulation1/1_schwarz_mit_Deckel/Signal Builder4 ==
  Demux : Demux  Tag=STV Demux  Outputs=6
      settings: DisplayOption=none
  FromWs : FromWorkspace  Tag=STV FromWs  VariableName=tuvar
      SigBuilderData=|
      | common.afterFinalStr = 'Extrapolate'
      | common.sampleTime = 0
      | dataSet.timeRange = [0 11]
      | dataSet.name = 'Group 1'
      | sbobj.Groups.Name = 'Group 1'
      | sbobj.Groups.Signals(1).Name = 'zylinder_platziert'
      | sbobj.Groups.Signals(1).XData = [0 0.3 0.3 11]
      | sbobj.Groups.Signals(1).YData = [1 1 0 0]
      | sbobj.Groups.Signals(2).Name = 'zylinder_schwarz'
      | sbobj.Groups.Signals(2).XData = [0 5.6 5.6 11]
      | sbobj.Groups.Signals(2).YData = [1 1 0 0]
      | sbobj.Groups.Signals(3).Name = 'zylinder_hoehe'
      | sbobj.Groups.Signals(3).XData = [0 5 5 5.6 5.6 11]
      | sbobj.Groups.Signals(3).YData = [0 0 25 25 0 0]
      | sbobj.Groups.Signals(4).Name = 'arbeitsraum_frei'
      | sbobj.Groups.Signals(4).XData = [0 0.5 0.5 10.5 10.5 10.8 10.8 11]
      | sbobj.Groups.Signals(4).YData = [1 1 0 0 1 1 0 0]
      | sbobj.Groups.Signals(5).Name = 'zylinder_entfernt_folge'
      | sbobj.Groups.Signals(5).XData = [0 10 10 10.5 10.5 11]
      | sbobj.Groups.Signals(5).YData = [0 0 1 1 0 0]
      | sbobj.Groups.Signals(6).Name = 'folge_belegt'
      | sbobj.Groups.Signals(6).XData = [0 4 4 5.5 5.5 11]
      | sbobj.Groups.Signals(6).YData = [0 0 1 1 0 0]
      | sbobj.Groups.TimeRange = [0 11]
  zylinder_platziert : Outport  Tag=STV Outport  VectorParamsAs1DForOutWhenUnconnected=off
  zylinder_schwarz : Outport  Tag=STV Outport  Port=2  VectorParamsAs1DForOutWhenUnconnected=off
  zylinder_hoehe : Outport  Tag=STV Outport  Port=3  VectorParamsAs1DForOutWhenUnconnected=off
  arbeitsraum_frei : Outport  Tag=STV Outport  Port=4  VectorParamsAs1DForOutWhenUnconnected=off
  zylinder_entfernt_folge : Outport  Tag=STV Outport  Port=5  VectorParamsAs1DForOutWhenUnconnected=off
  folge_belegt : Outport  Tag=STV Outport  Port=6  VectorParamsAs1DForOutWhenUnconnected=off
  wires:
  Demux/1 -> zylinder_platziert/1
  FromWs/1 -> Demux/1
  Demux/2 -> zylinder_schwarz/1
  Demux/3 -> zylinder_hoehe/1
  Demux/4 -> arbeitsraum_frei/1
  Demux/5 -> zylinder_entfernt_folge/1
  Demux/6 -> folge_belegt/1

== system Vorlage_Anlagenteil_Pruefen_Jaehocha/Systemtest Simulation1/1_schwarz_mit_Deckel/arbeitsraum_frei ==
  Add : Sum  Inputs=++++
  Constant : Constant
  Constant1 : Constant  Value=-1
  Constant2 : Constant
  Constant3 : Constant  Value=-1
  Data Type Conversion : DataTypeConversion  OutDataTypeStr=boolean
  Delay : Delay  DelayLength=0
  Delay1 : Delay  DelayLength=200
  Delay2 : Delay  DelayLength=1050
  Delay3 : Delay  DelayLength=1080
  Out1 : Outport  VectorParamsAs1DForOutWhenUnconnected=off
  wires:
  Constant/1 -> Delay/1
  Constant1/1 -> Delay1/1
  Delay/1 -> Add/1
  Delay1/1 -> Add/2
  Add/1 -> Data Type Conversion/1
  Data Type Conversion/1 -> Out1/1
  Constant2/1 -> Delay2/1
  Delay2/1 -> Add/3
  Constant3/1 -> Delay3/1
  Delay3/1 -> Add/4

== system Vorlage_Anlagenteil_Pruefen_Jaehocha/Systemtest Simulation1/1_schwarz_mit_Deckel/aufzug_abwaerts ==
  Add : Sum
  Constant : Constant
  Constant1 : Constant  Value=-1
  Data Type Conversion : DataTypeConversion  OutDataTypeStr=boolean
  Delay : Delay  DelayLength=600
  Delay1 : Delay  DelayLength=1050
  Out1 : Outport  VectorParamsAs1DForOutWhenUnconnected=off
  wires:
  Constant/1 -> Delay/1
  Constant1/1 -> Delay1/1
  Delay/1 -> Add/1
  Delay1/1 -> Add/2
  Add/1 -> Data Type Conversion/1
  Data Type Conversion/1 -> Out1/1

== system Vorlage_Anlagenteil_Pruefen_Jaehocha/Systemtest Simulation1/1_schwarz_mit_Deckel/aufzug_aufwaerts ==
  Add : Sum
  Constant : Constant
  Constant1 : Constant  Value=-1
  Data Type Conversion : DataTypeConversion  OutDataTypeStr=boolean
  Delay : Delay  DelayLength=50
  Delay1 : Delay  DelayLength=500
  Out1 : Outport  VectorParamsAs1DForOutWhenUnconnected=off
  wires:
  Constant/1 -> Delay/1
  Constant1/1 -> Delay1/1
  Delay/1 -> Add/1
  Delay1/1 -> Add/2
  Add/1 -> Data Type Conversion/1
  Data Type Conversion/1 -> Out1/1

== system Vorlage_Anlagenteil_Pruefen_Jaehocha/Systemtest Simulation1/1_schwarz_mit_Deckel/done_signal ==
  Constant : Constant
  Data Type Conversion : DataTypeConversion  OutDataTypeStr=boolean
  Delay : Delay  DelayLength=1080
  Out1 : Outport  VectorParamsAs1DForOutWhenUnconnected=off
  wires:
  Constant/1 -> Delay/1
  Data Type Conversion/1 -> Out1/1
  Delay/1 -> Data Type Conversion/1

== system Vorlage_Anlagenteil_Pruefen_Jaehocha/Systemtest Simulation1/1_schwarz_mit_Deckel/folge_belegt ==
  Add : Sum
  Constant1 : Constant
  Constant2 : Constant  Value=-1
  Data Type Conversion1 : DataTypeConversion  OutDataTypeStr=boolean
  Delay : Delay  DelayLength=400
  Delay1 : Delay  DelayLength=550
  Out1 : Outport  VectorParamsAs1DForOutWhenUnconnected=off
  wires:
  Data Type Conversion1/1 -> Out1/1
  Constant1/1 -> Delay/1
  Constant2/1 -> Delay1/1
  Delay/1 -> Add/1
  Delay1/1 -> Add/2
  Add/1 -> Data Type Conversion1/1

== system Vorlage_Anlagenteil_Pruefen_Jaehocha/Systemtest Simulation1/1_schwarz_mit_Deckel/luft_an ==
  Add : Sum
  Constant : Constant
  Constant1 : Constant  Value=-1
  Data Type Conversion : DataTypeConversion  OutDataTypeStr=boolean
  Delay : Delay  DelayLength=550
  Delay1 : Delay  DelayLength=750
  Out1 : Outport  VectorParamsAs1DForOutWhenUnconnected=off
  wires:
  Constant/1 -> Delay/1
  Constant1/1 -> Delay1/1
  Delay/1 -> Add/1
  Delay1/1 -> Add/2
  Add/1 -> Data Type Conversion/1
  Data Type Conversion/1 -> Out1/1

== system Vorlage_Anlagenteil_Pruefen_Jaehocha/Systemtest Simulation1/1_schwarz_mit_Deckel/out5 ==
  Add : Sum
  Constant : Constant
  Constant1 : Constant  Value=-1
  Data Type Conversion : DataTypeConversion  OutDataTypeStr=boolean
  Delay : Delay  DelayLength=0
  Delay1 : Delay  DelayLength=0
  Out1 : Outport  VectorParamsAs1DForOutWhenUnconnected=off
  wires:
  Constant/1 -> Delay/1
  Constant1/1 -> Delay1/1
  Delay/1 -> Add/1
  Delay1/1 -> Add/2
  Add/1 -> Data Type Conversion/1
  Data Type Conversion/1 -> Out1/1

== system Vorlage_Anlagenteil_Pruefen_Jaehocha/Systemtest Simulation1/1_schwarz_mit_Deckel/out6 ==
  Add : Sum
  Constant : Constant
  Constant1 : Constant  Value=-1
  Data Type Conversion : DataTypeConversion  OutDataTypeStr=boolean
  Delay : Delay  DelayLength=0
  Delay1 : Delay  DelayLength=0
  Out1 : Outport  VectorParamsAs1DForOutWhenUnconnected=off
  wires:
  Constant/1 -> Delay/1
  Constant1/1 -> Delay1/1
  Delay/1 -> Add/1
  Delay1/1 -> Add/2
  Add/1 -> Data Type Conversion/1
  Data Type Conversion/1 -> Out1/1

== system Vorlage_Anlagenteil_Pruefen_Jaehocha/Systemtest Simulation1/1_schwarz_mit_Deckel/out7 ==
  Add : Sum
  Constant : Constant
  Constant1 : Constant  Value=-1
  Data Type Conversion : DataTypeConversion  OutDataTypeStr=boolean
  Delay : Delay  DelayLength=0
  Delay1 : Delay  DelayLength=0
  Out1 : Outport  VectorParamsAs1DForOutWhenUnconnected=off
  wires:
  Constant/1 -> Delay/1
  Constant1/1 -> Delay1/1
  Delay/1 -> Add/1
  Delay1/1 -> Add/2
  Add/1 -> Data Type Conversion/1
  Data Type Conversion/1 -> Out1/1

== system Vorlage_Anlagenteil_Pruefen_Jaehocha/Systemtest Simulation1/1_schwarz_mit_Deckel/station_frei ==
  Add : Sum
  Constant : Constant
  Constant1 : Constant  Value=-1
  Data Type Conversion : DataTypeConversion  OutDataTypeStr=boolean
  Delay : Delay  DelayLength=0
  Delay1 : Delay  DelayLength=10
  Out1 : Outport  VectorParamsAs1DForOutWhenUnconnected=off
  wires:
  Constant/1 -> Delay/1
  Constant1/1 -> Delay1/1
  Delay/1 -> Add/1
  Delay1/1 -> Add/2
  Add/1 -> Data Type Conversion/1
  Data Type Conversion/1 -> Out1/1

== system Vorlage_Anlagenteil_Pruefen_Jaehocha/Systemtest Simulation1/1_schwarz_mit_Deckel/zylinder_ausschieben ==
  Add : Sum
  Constant : Constant
  Constant1 : Constant  Value=-1
  Data Type Conversion : DataTypeConversion  OutDataTypeStr=boolean
  Delay : Delay  DelayLength=550
  Delay1 : Delay  DelayLength=620
  Out1 : Outport  VectorParamsAs1DForOutWhenUnconnected=off
  wires:
  Constant/1 -> Delay/1
  Constant1/1 -> Delay1/1
  Delay/1 -> Add/1
  Delay1/1 -> Add/2
  Add/1 -> Data Type Conversion/1
  Data Type Conversion/1 -> Out1/1

== system Vorlage_Anlagenteil_Pruefen_Jaehocha/Systemtest Simulation1/1_schwarz_mit_Deckel/zylinder_entfernt_folge ==
  Add : Sum
  Constant : Constant
  Constant1 : Constant  Value=-1
  Data Type Conversion : DataTypeConversion  OutDataTypeStr=boolean
  Delay : Delay  DelayLength=1000
  Delay1 : Delay  DelayLength=1050
  Out1 : Outport  VectorParamsAs1DForOutWhenUnconnected=off
  wires:
  Constant/1 -> Delay/1
  Constant1/1 -> Delay1/1
  Delay/1 -> Add/1
  Delay1/1 -> Add/2
  Add/1 -> Data Type Conversion/1
  Data Type Conversion/1 -> Out1/1

== system Vorlage_Anlagenteil_Pruefen_Jaehocha/Systemtest Simulation1/1_schwarz_mit_Deckel/zylinder_hoehe ==
  Add : Sum
  Constant : Constant  Value=25
  Constant1 : Constant  Value=-25
  Delay : Delay  DelayLength=50
  Delay1 : Delay  DelayLength=900
  Out1 : Outport  VectorParamsAs1DForOutWhenUnconnected=off
  wires:
  Constant/1 -> Delay/1
  Constant1/1 -> Delay1/1
  Delay/1 -> Add/1
  Delay1/1 -> Add/2
  Add/1 -> Out1/1

== system Vorlage_Anlagenteil_Pruefen_Jaehocha/Systemtest Simulation1/1_schwarz_mit_Deckel/zylinder_platziert ==
  Add : Sum
  Constant : Constant
  Constant1 : Constant  Value=-1
  Data Type Conversion : DataTypeConversion  OutDataTypeStr=boolean
  Delay : Delay  DelayLength=50
  Delay1 : Delay  DelayLength=70
  Out1 : Outport  VectorParamsAs1DForOutWhenUnconnected=off
  wires:
  Constant/1 -> Delay/1
  Constant1/1 -> Delay1/1
  Delay/1 -> Add/1
  Delay1/1 -> Add/2
  Add/1 -> Data Type Conversion/1
  Data Type Conversion/1 -> Out1/1

== system Vorlage_Anlagenteil_Pruefen_Jaehocha/Systemtest Simulation1/1_schwarz_mit_Deckel/zylinder_schwarz ==
  Add : Sum
  Constant : Constant
  Constant1 : Constant  Value=-1
  Data Type Conversion : DataTypeConversion  OutDataTypeStr=boolean
  Delay : Delay  DelayLength=0
  Delay1 : Delay  DelayLength=700
  Out1 : Outport  VectorParamsAs1DForOutWhenUnconnected=off
  wires:
  Constant/1 -> Delay/1
  Constant1/1 -> Delay1/1
  Delay/1 -> Add/1
  Delay1/1 -> Add/2
  Add/1 -> Data Type Conversion/1
  Data Type Conversion/1 -> Out1/1
